simulink model "IEX_NOMremoval"  (Simulink 8.5)
settings: Solver=ode15s  StartTime=0.0  StopTime=700*24*3600  RelTol=1e-3
undefined symbols (not defined in the file): B, U, x0
settings Model: Creator=psross  LastModifiedBy=Martijn  ExtModeTrigMode=oneshot  ExtModeArmWhenConnect=off
settings DataIOCC: LimitDataPoints=off  SignalLoggingName=sigsOut
settings OptimizationCC: BooleanDataType=off  InitFltsAndDblsToZero=on
settings DebuggingCC: SaveWithParameterizedLinksMsg=none  SignalResolutionControl=TryResolveAllWithWarning  MultiTaskDSMMsg=warning  MultiTaskCondExecSysMsg=none  FcnCallInpInsideContextMsg=UseLocalSettings  StrictBusMsg=None
settings HardwareCC: TargetUnknown=on

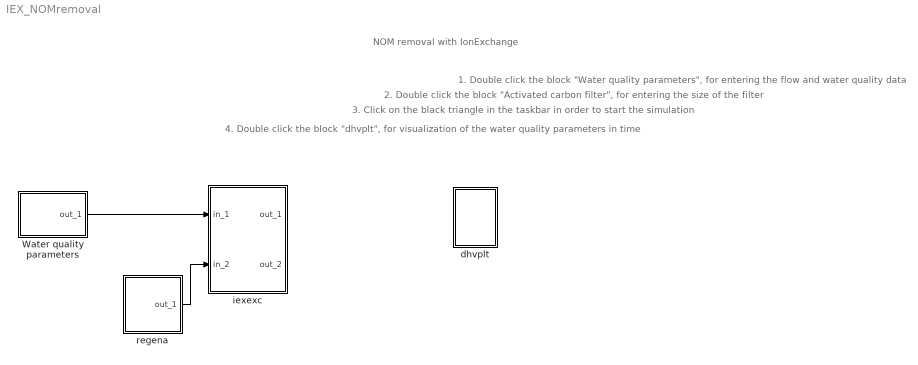
== system IEX_NOMremoval ==
  note: NOM removal with IonExchange
  note: 2. Double click the block "Activated carbon filter", for entering the size of the filter
  note: 3. Click on the black triangle in the taskbar in order to start the simulation
  note: 1. Double click the block "Water quality parameters", for entering the flow and water quality data
  note: 4. Double click the block "dhvplt", for visualization of the water quality parameters in time
  Water quality parameters : Subsystem  Description=The water flow and the water quality data must be filled out in the 'Water quality parameters' block. Each project must start with a 'Water quality parameters' block.
      mask init:
      | filenaam='./StimelaData/rawwater.mat';
      | 
      | [Pn,Fn,Fext]=Fileprop(filenaam);
      | 
      | errstr = st_UniqName(filenaam,'filenaam=''','SubSystem','OpenFcn');
      | if errstr, error([errstr 'The filename "' filenaam '" is already in use. Choose a different filename.']), end
      | 
      | P = invruw_p(filenaam);
      | [B,x0,U]=invruw_i(filenaam);
      settings: OpenFcn=|
      | filenaam='./StimelaData/rawwater.mat';
      | st_ParameterInput('init',gcb,filenaam,'invruw');
      mask Display:
      | plot(0,0,100,100,[80 100],[ 50 50],[80 100],[ 55 55],[20 80 80 20 20],[10 10 90  90 10]);
      | disp('')
      | text(50,50,'invruw', 'horizontalAlignment', 'center', 'verticalAlignment', 'middle');
      | text(50,0,Fn, 'horizontalAlignment', 'center', 'verticalAlignment', 'base');
  dhvplt : Subsystem
      settings: OpenFcn=plotStimela2
      mask Display:
      | plot(0,0,100,100,[80,20,20],[20,20,80],[80,69,60,52,45,39,33,28,24,20],[65,65,64,61,57,52,45,37,30,20])
      | disp('');
      | text(100,100,'Stimela', 'horizontalAlignment', 'right', 'verticalAlignment', 'top');
  iexexc : Subsystem  Description="This model calculates the removal of DOC with an activated carbon filter. Make sure the length of a filterrun is bigger than the simulation stop time entered in \"Parameters...\" on the \"Simulation\" menu."
      mask init:
      | filenaam='./StimelaData/ionexchange.mat';
      | 
      | [Pn,Fn,Fext]=Fileprop(filenaam);
      | 
      | errstr = st_UniqName(filenaam,'filenaam=''','SubSystem','OpenFcn');
      | if errstr, error([errstr 'The filename "' filenaam '" is already in use. Choose a different filename.']), end
      | 
      | P = iexexc_p(filenaam);
      | [B,x0,U]=iexexc_i(filenaam);
      settings: OpenFcn=|
      | filenaam='./StimelaData/ionexchange.mat';
      | st_ParameterInput('init',gcb,filenaam,'iexexc');
      mask Display:
      | plot(0,0,100,100,[25.000000,25.000000,75.000000,75.000000,87.500000],[75.000000,25.000000,25.000000,30.000000,30.000000],[87.500000,75.000000,75.000000],[37.500000,37.500000,75.000000],[25.000000,75.000000],[65.000000,65.000000],[25.000000,75.000000],[42.500000,42.500000],[37.500000,42.500000],[52.500000,52.500000],[50.000000,55.000000],[52.500000,52.500000],[62.500000,67.500000],[52.500000,52.500000])
      | disp('')
      | text(50,50,'iexexc', 'horizontalAlignment', 'center', 'verticalAlignment', 'middle');
      | text(50,0,Fn, 'horizontalAlignment', 'center', 'verticalAlignment', 'base');
  regena : Subsystem  Description=During a simulation the filter can be backwashed with the backwash module, so a number of successive filterruns can be simulated.
      mask init:
      | filenaam='./StimelaData/regeneration.mat';
      | 
      | [Pn,Fn,Fext]=Fileprop(filenaam);
      | 
      | errstr = st_UniqName(filenaam,'filenaam=''','SubSystem','OpenFcn');
      | if errstr, error([errstr 'The filename "' filenaam '" is already in use. Choose a different filename.']), end
      | 
      | P = regena_p(filenaam);
      | [B,x0,U]=regena_i(filenaam);
      settings: OpenFcn=|
      | filenaam='./StimelaData/regeneration.mat';
      | st_ParameterInput('init',gcb,filenaam,'regena');
      mask Display:
      | plot(0,0,100,100,[80,80,20,20],[80,20,20,80],[40,42,38,40,40],[70,67,67,70,30],[60,62,58,60,60],[70,67,67,70,30]);
      | disp('')
      | text(50,50,'regena', 'horizontalAlignment', 'center', 'verticalAlignment', 'middle');
      | text(50,0,Fn, 'horizontalAlignment', 'center', 'verticalAlignment', 'base');
  wires:
  Water quality parameters/1(out_1) -> iexexc/1(in_1)
  regena/1(out_1) -> iexexc/2(in_2)

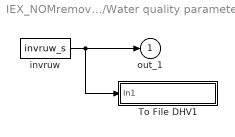
== system IEX_NOMremoval/Water quality parameters ==
  To File DHV1 : Subsystem  mask(To File DHV){naam=[filenaam(1:length(filenaam)-4) '_out.sti']}
      mask prompts: naam "Naam van bestand"
      mask init:
      | set_param([gcb '/To File'],'Filename',naam);
      mask Display: disp(naam)
  invruw : S-Function  FunctionName=invruw_s  Parameters=B,x0,U,P
  out_1 : Outport  InitialOutput=0
  wires:
  invruw/1 -> out_1/1, To File DHV1/1(In1)

== system IEX_NOMremoval/dhvplt ==
  note: plotten

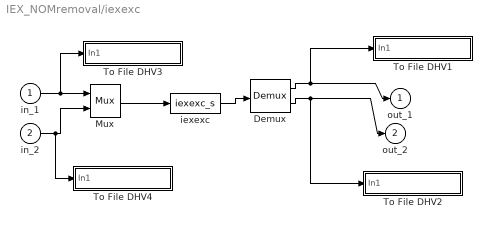
== system IEX_NOMremoval/iexexc ==
  in_1 : Inport
  in_2 : Inport  Port=2
  Demux : Demux  Outputs=[U.Number B.Measurements]
  Mux : Mux  Inputs=[U.Number B.Setpoints]
  To File DHV1 : Subsystem  mask(To File DHV){naam=[filenaam(1:length(filenaam)-4) '_out.sti']}
      mask prompts: naam "Naam van bestand"
      mask init:
      | set_param([gcb '/To File'],'Filename',naam);
      mask Display: disp(naam)
  To File DHV2 : Subsystem  mask(To File DHV){naam=[filenaam(1:length(filenaam)-4) '_EM.sti']}
      mask prompts: naam "Naam van bestand"
      mask init:
      | set_param([gcb '/To File'],'Filename',naam);
      mask Display: disp(naam)
  To File DHV3 : Subsystem  mask(To File DHV){naam=[filenaam(1:length(filenaam)-4) '_in.sti']}
      mask prompts: naam "Naam van bestand"
      mask init:
      | set_param([gcb '/To File'],'Filename',naam);
      mask Display: disp(naam)
  To File DHV4 : Subsystem  mask(To File DHV){naam=[filenaam(1:length(filenaam)-4) '_ES.sti']}
      mask prompts: naam "Naam van bestand"
      mask init:
      | set_param([gcb '/To File'],'Filename',naam);
      mask Display: disp(naam)
  iexexc : S-Function  FunctionName=iexexc_s  Parameters=B,x0,U,P
  out_1 : Outport  InitialOutput=0
  out_2 : Outport  Port=2  InitialOutput=0
  wires:
  in_2/1 -> To File DHV4/1(In1), Mux/2
  Mux/1 -> iexexc/1
  in_1/1 -> To File DHV3/1(In1), Mux/1
  iexexc/1 -> Demux/1
  Demux/1 -> To File DHV1/1(In1), out_1/1
  Demux/2 -> To File DHV2/1(In1), out_2/1

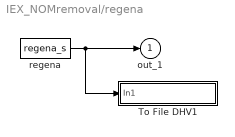
== system IEX_NOMremoval/regena ==
  To File DHV1 : Subsystem  mask(To File DHV){naam=[filenaam(1:length(filenaam)-4) '_out.sti']}
      mask prompts: naam "Naam van bestand"
      mask init:
      | set_param([gcb '/To File'],'Filename',naam);
      mask Display: disp(naam)
  regena : S-Function  FunctionName=regena_s  Parameters=B,x0,U,P
  out_1 : Outport  InitialOutput=0
  wires:
  regena/1 -> To File DHV1/1(In1), out_1/1

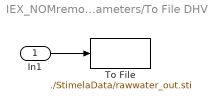
== system IEX_NOMremoval/Water quality parameters/To File DHV1 ==
  In1 : Inport
  To File : ToFile  Filename=./StimelaData/rawwater_out.sti  MatrixName=invruwout
  wires:
  In1/1 -> To File/1

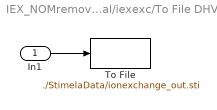
== system IEX_NOMremoval/iexexc/To File DHV1 ==
  In1 : Inport
  To File : ToFile  Filename=./StimelaData/ionexchange_out.sti  MatrixName=iexexcout
  wires:
  In1/1 -> To File/1

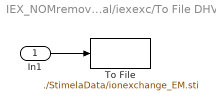
== system IEX_NOMremoval/iexexc/To File DHV2 ==
  In1 : Inport
  To File : ToFile  Filename=./StimelaData/ionexchange_EM.sti  MatrixName=iexexcEM
  wires:
  In1/1 -> To File/1

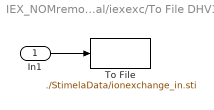
== system IEX_NOMremoval/iexexc/To File DHV3 ==
  In1 : Inport
  To File : ToFile  Filename=./StimelaData/ionexchange_in.sti  MatrixName=iexexcin
  wires:
  In1/1 -> To File/1

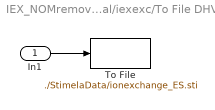
== system IEX_NOMremoval/iexexc/To File DHV4 ==
  In1 : Inport
  To File : ToFile  Filename=./StimelaData/ionexchange_ES.sti  MatrixName=iexexcES
  wires:
  In1/1 -> To File/1

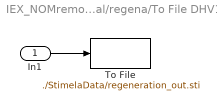
== system IEX_NOMremoval/regena/To File DHV1 ==
  In1 : Inport
  To File : ToFile  Filename=./StimelaData/regeneration_out.sti  MatrixName=regenaout
  wires:
  In1/1 -> To File/1
